simulink model "Battery_v1"  (R2024b)
settings: Solver=VariableStepAuto  StartTime=0.0  StopTime=inf  RelTol=1e-3
settings Model: Creator=miche  LastModifiedBy=miche

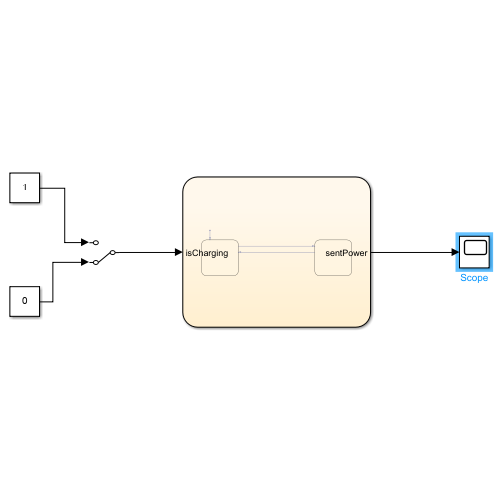
[thumbnail: Simulink's stored preview of the top-level diagram]
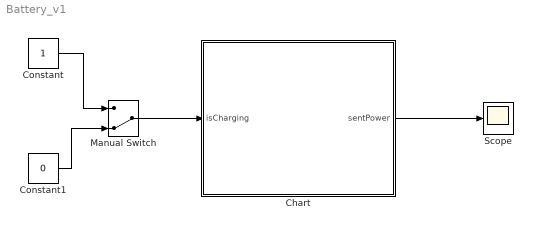
== system Battery_v1 ==
  Chart : Stateflow chart  TreatAsAtomicUnit=on
  Constant : Constant  SampleTime=0.5
  Constant1 : Constant  Value=0  SampleTime=0.5
  Manual Switch : ManualSwitch  CurrentSetting=0
  Scope : Scope
  wires:
  Constant/1 -> Manual Switch/1
  Constant1/1 -> Manual Switch/2
  Manual Switch/1 -> Chart/1(isCharging)
  Chart/1(sentPower) -> Scope/1

== stateflow chart Battery_v1/Chart ==
  state Charge
    entry:
    sentPower = 0;
    during:
    charge = charge+4;
  state Discharge
    entry:
    sentPower = 3.5;
    during:
    charge=charge-3;
  (default) -> Charge
  Charge -> Discharge : [~isCharging]
  Discharge -> Charge : [isCharging]
  data: isCharging input; sentPower output; charge local =50
